simulink model "building_PHPP_v1"  (R2018b)
settings: Solver=ode23s  StartTime=-building.preruntime+8760*3600  StopTime=building.runtime+8760*3600  EnableMultiTasking=on
StartFcn:
  | tic
StopFcn:
  | toc
values from neighbouring files (symbols this model uses):
  A = 7*10*2    (= 140)    [theta_ground_v1.m]    (also in xlswrite1.m = num2cell(data))
  B = A/(0.5 * P)    (= 8.23529411765)    [theta_ground_v1.m]
  building = obj    [BUILDING.m]    (also in create_building_automatic.m = building.save(); ini_building_automatic.m = building.add_variant_hvac(building.variant_hvac, hvac); load_building_automatic.m = building.save())
  C = zeros(1,length(d)+1)    [CONSTRUCTION.m]    (also in DOOR.m = [0 0 0]; WALL.m = [0 0 0]; WINDOW.m = [0 0 0])
  cp = str2num(value)    [CONSTRUCTION.m]
  p = [timevec_weather weather(:,12)]    [BOUNDARY.m]    (also in WEATHER.m = 0; init_carnotUIBK.m = cell2mat(carnotUIBKpaths(i,2)))
  rho = str2num(value)    [CONSTRUCTION.m]    (also in theta_ground_v1.m = 2000)
undefined symbols (not defined in the file or in its folder): Dd, Dreifach, get_building, Qdot_C, Qdot_C_energy, Qdot_H, Qdot_H_energy, Qdot_I_electricity, Qdot_I_electricity_energy, Qdot_I_light, Qdot_I_light_energy, Qdot_I_person, Qdot_I_person_energy, Qdot_S, Qdot_S_energy, Qdot_T_ground, Qdot_T_ground_energy, Qdot_T_neighbour, Qdot_T_neighbour_energy, Qdot_T_opaque, Qdot_T_opaque_energy, Qdot_T_window, Qdot_T_window_energy, Qdot_V_infiltration, Qdot_V_infiltration_energy, Qdot_V_mech, Qdot_V_mech_energy, Qdot_V_window, Qdot_V_window_energy, Tc, Tr, Ts, Wärmeschutzglas, x_CO2, x_H2O, x_VOC
libraries: carnotUIBK x1874, carnot x5, simulink x3
(part 2 of 34)

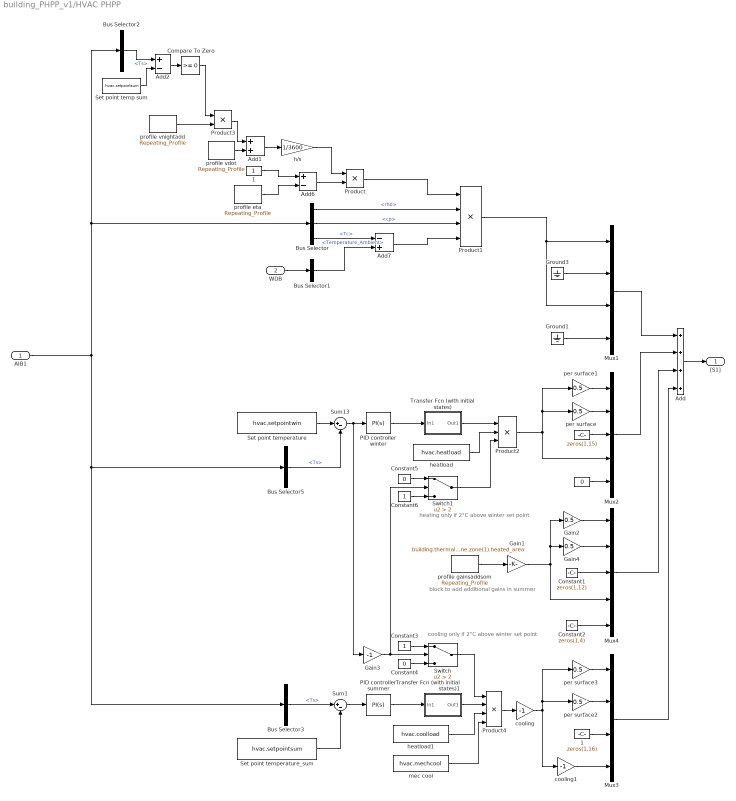
== system building_PHPP_v1/HVAC PHPP ==
  note: cooling only if 2°C above winter set point
  note: block to add additional gains in summer
  note: heating only if 2°C above winter set point
  AIB1 : Inport
  WDB : Inport  Port=2
  " " : Constant  Value=0
  "   " : Constant  Value=zeros(1,15)
  "   1" : Constant  Value=zeros(1,16)
  1 : Constant
  Add : Sum  Inputs=++++
  Add1 : Sum
  Add2 : Sum  Inputs=+-
  Add6 : Sum  Inputs=+-
  Add7 : Sum  Inputs=-+
  Bus Selector : BusSelector  OutputSignals=rho,cp,Tc
  Bus Selector1 : BusSelector  OutputSignals=Temperature_Ambient
  Bus Selector2 : BusSelector  OutputSignals=Ts
  Bus Selector3 : BusSelector  OutputSignals=Ts
  Bus Selector5 : BusSelector  OutputSignals=Ts
  Compare To Zero : simulink/Logic and Bit Operations/Compare To Zero  relop=>=  OutDataTypeStr=boolean
  Constant1 : Constant  Value=zeros(1,12)
  Constant2 : Constant  Value=zeros(1,4)
  Constant3 : Constant
  Constant4 : Constant  Value=0
  Constant5 : Constant  Value=0
  Constant6 : Constant
  Gain1 : Gain  Gain=building.thermalzone.zone(1).heated_area  SaturateOnIntegerOverflow=on  OutDataTypeStr=Inherit: Same as input  ParamDataTypeStr=Inherit: Same as input
  Gain2 : Gain  Gain=0.5  SaturateOnIntegerOverflow=on  OutDataTypeStr=Inherit: Same as input  ParamDataTypeStr=Inherit: Same as input
  Gain3 : Gain  Gain=-1  SaturateOnIntegerOverflow=on  OutDataTypeStr=Inherit: Same as input  ParamDataTypeStr=Inherit: Same as input
  Gain4 : Gain  Gain=0.5  SaturateOnIntegerOverflow=on  OutDataTypeStr=Inherit: Same as input  ParamDataTypeStr=Inherit: Same as input
  Ground1 : Ground
  Ground3 : Ground
  Mux1 : Mux  Inputs=[1 10 1 7]
  Mux2 : Mux  Inputs=[1 1 15 1 1]
  Mux3 : Mux  Inputs=[1 1 16 1]
  Mux4 : Mux  Inputs=[1 1 12 1 4]
  PID controller summer : simulink/Continuous/PID Controller  Controller=PI  Form=Ideal  TimeDomain=Continuous-time  SampleTime=-1  IntegratorMethod=Forward Euler  FilterMethod=Forward Euler  ControllerParametersSource=internal  P=hvac.valves.Kp  I=(1/(hvac.valves.Tn*60))  D=0  UseFilter=on  N=100  TunerSelectOption=Transfer Function Based (PID Tuner App)  InitialConditionSource=internal  InitialConditionForIntegrator=0  InitialConditionForFilter=0  DifferentiatorICPrevScaledInput=0  ExternalReset=none  TrackingMode=off  Kt=1  LimitOutput=on  UpperSaturationLimit=hvac.valves.valve_up  LowerSaturationLimit=hvac.valves.valve_low  LinearizeAsGain=off  AntiWindupMode=clamping  Kb=1  POutMin=[]  POutMax=[]  IOutMin=[]  IOutMax=[]  DOutMin=[]  DOutMax=[]  NOutMin=[]  NOutMax=[]  SumOutMin=[]  SumOutMax=[]  SaturationOutMin=[]  SaturationOutMax=[]  PParamMin=[]  PParamMax=[]  IParamMin=[]  IParamMax=[]  DParamMin=[]  DParamMax=[]  NParamMin=[]  NParamMax=[]  KbParamMin=[]  KbParamMax=[]  KtParamMin=[]  KtParamMax=[]  KbOutMin=[]  KbOutMax=[]  KtOutMin=[]  KtOutMax=[]  IntegratorOutMin=[]  IntegratorOutMax=[]  FilterOutMin=[]  FilterOutMax=[]  SumI1OutMin=[]  SumI1OutMax=[]  SumI2OutMin=[]  SumI2OutMax=[]  SumI3OutMin=[]  SumI3OutMax=[]  SumI4OutMin=[]  SumI4OutMax=[]  SumDOutMin=[]  SumDOutMax=[]  DifferentiatorOutMin=[]  DifferentiatorOutMax=[]  FilterDiffOutCoefMin=[]  FilterDiffOutCoefMax=[]  ReciprocalOutMin=[]  ReciprocalOutMax=[]  SumDenOutMin=[]  SumDenOutMax=[]  SumNumOutMin=[]  SumNumOutMax=[]  DivideOutMin=[]  DivideOutMax=[]  IntegratorContinuousStateAttributes=''  IntegratorStateMustResolveToSignalObject=off  IntegratorRTWStateStorageClass=Auto  FilterContinuousStateAttributes=''  FilterStateMustResolveToSignalObject=off  FilterRTWStateStorageClass=Auto  ParallelPVariant=Passthrough  IdealPVariant=InternalParameters  IVariant=InternalParameters  DVariant=Disabled  IntegratorVariant=Continuous  SatVariant=Enabled  AWVariant=ContClampingIdeal  PCopyVariant=InternalParamsIdeal  TRVariant=Disabled  FdbkBlocksVariant=Forward  IdealPFdbkVariant=Disabled  SatFdbkVariant=Disabled  DerivativeFilterVariant=Disabled  NVariant=Disabled  NCopyVariant=Disabled_SignalSpec  FilterICVariant=Disabled  IntegratorICVariant=InternalICs  ExternalResetVariant=Disabled  TRSumVariant=Passthrough  SumFdbkVariant=Disabled  SumVariant=Sum_PI
  PID controller winter : simulink/Continuous/PID Controller  Controller=PI  Form=Ideal  TimeDomain=Continuous-time  SampleTime=-1  IntegratorMethod=Forward Euler  FilterMethod=Forward Euler  ControllerParametersSource=internal  P=hvac.valves.Kp  I=(1/(hvac.valves.Tn*60))  D=0  UseFilter=on  N=100  TunerSelectOption=Transfer Function Based (PID Tuner App)  InitialConditionSource=internal  InitialConditionForIntegrator=0  InitialConditionForFilter=0  DifferentiatorICPrevScaledInput=0  ExternalReset=none  TrackingMode=off  Kt=1  LimitOutput=on  UpperSaturationLimit=hvac.valves.valve_up  LowerSaturationLimit=hvac.valves.valve_low  LinearizeAsGain=off  AntiWindupMode=clamping  Kb=1  POutMin=[]  POutMax=[]  IOutMin=[]  IOutMax=[]  DOutMin=[]  DOutMax=[]  NOutMin=[]  NOutMax=[]  SumOutMin=[]  SumOutMax=[]  SaturationOutMin=[]  SaturationOutMax=[]  PParamMin=[]  PParamMax=[]  IParamMin=[]  IParamMax=[]  DParamMin=[]  DParamMax=[]  NParamMin=[]  NParamMax=[]  KbParamMin=[]  KbParamMax=[]  KtParamMin=[]  KtParamMax=[]  KbOutMin=[]  KbOutMax=[]  KtOutMin=[]  KtOutMax=[]  IntegratorOutMin=[]  IntegratorOutMax=[]  FilterOutMin=[]  FilterOutMax=[]  SumI1OutMin=[]  SumI1OutMax=[]  SumI2OutMin=[]  SumI2OutMax=[]  SumI3OutMin=[]  SumI3OutMax=[]  SumI4OutMin=[]  SumI4OutMax=[]  SumDOutMin=[]  SumDOutMax=[]  DifferentiatorOutMin=[]  DifferentiatorOutMax=[]  FilterDiffOutCoefMin=[]  FilterDiffOutCoefMax=[]  ReciprocalOutMin=[]  ReciprocalOutMax=[]  SumDenOutMin=[]  SumDenOutMax=[]  SumNumOutMin=[]  SumNumOutMax=[]  DivideOutMin=[]  DivideOutMax=[]  IntegratorContinuousStateAttributes=''  IntegratorStateMustResolveToSignalObject=off  IntegratorRTWStateStorageClass=Auto  FilterContinuousStateAttributes=''  FilterStateMustResolveToSignalObject=off  FilterRTWStateStorageClass=Auto  ParallelPVariant=Passthrough  IdealPVariant=InternalParameters  IVariant=InternalParameters  DVariant=Disabled  IntegratorVariant=Continuous  SatVariant=Enabled  AWVariant=ContClampingIdeal  PCopyVariant=InternalParamsIdeal  TRVariant=Disabled  FdbkBlocksVariant=Forward  IdealPFdbkVariant=Disabled  SatFdbkVariant=Disabled  DerivativeFilterVariant=Disabled  NVariant=Disabled  NCopyVariant=Disabled_SignalSpec  FilterICVariant=Disabled  IntegratorICVariant=InternalICs  ExternalResetVariant=Disabled  TRSumVariant=Passthrough  SumFdbkVariant=Disabled  SumVariant=Sum_PI
  Product : Product
  Product1 : Product  Inputs=4
  Product2 : Product  Inputs=3
  Product3 : Product
  Product4 : Product  Inputs=4
  Set point temp sum : Constant  Value=hvac.setpointsum  VectorParams1D=off
  Set point temperature : Constant  Value=hvac.setpointwin  VectorParams1D=off
  Set point temperature_sum : Constant  Value=hvac.setpointsum  VectorParams1D=off
  Sum1 : Sum  Inputs=|+-
  Sum13 : Sum  Inputs=|+-
  Switch : Switch  Criteria=u2 > Threshold  Threshold=2
  Switch1 : Switch  Criteria=u2 > Threshold  Threshold=2
  Transfer Fcn (with initial states) : Subsystem  mask(Transfer Function with Initial States){N=[1], D=[300  1], X0=0}
      mask prompts: N "Numerator:"; D "Denominator:"; X0 "Initial conditions:"
      mask help: Vector expressions for numerator, and denominator. Coefficients are in descending powers of s.
      mask init:
      | [A,B,C,Dd]=tf2ss(N,D);if (isempty(X0));[m,n]=size(A);X0=zeros(1,m); end;
      mask Help: Specify the initial states for the transfer function.  The state ordering is determined by the m-file tf2ss.  There is no unique mapping of the states in a transfer function to states in a state-space representation.  However, tf2ss will consistently use the same mapping for a given transfer function.
      mask Display: dpoly(N,D,'s')
  Transfer Fcn (with initial states)1 : Subsystem  mask(Transfer Function with Initial States){N=[1], D=[300  1], X0=0}
      mask prompts: N "Numerator:"; D "Denominator:"; X0 "Initial conditions:"
      mask help: Vector expressions for numerator, and denominator. Coefficients are in descending powers of s.
      mask init:
      | [A,B,C,Dd]=tf2ss(N,D);if (isempty(X0));[m,n]=size(A);X0=zeros(1,m); end;
      mask Help: Specify the initial states for the transfer function.  The state ordering is determined by the m-file tf2ss.  There is no unique mapping of the states in a transfer function to states in a state-space representation.  However, tf2ss will consistently use the same mapping for a given transfer function.
      mask Display: dpoly(N,D,'s')
  cooling : Gain  Gain=-1  SaturateOnIntegerOverflow=on  OutDataTypeStr=Inherit: Same as input  ParamDataTypeStr=Inherit: Same as input
  cooling1 : Gain  Gain=-1  SaturateOnIntegerOverflow=on  OutDataTypeStr=Inherit: Same as input  ParamDataTypeStr=Inherit: Same as input
  h/s : Gain  Gain=1/3600
  heatload : Constant  Value=hvac.heatload
  heatload1 : Constant  Value=hvac.coolload
  mec cool : Constant  Value=hvac.mechcool
  per surface{,1..3} (4 alike) : Gain  Gain=0.5  SaturateOnIntegerOverflow=on  OutDataTypeStr=Inherit: Same as input  ParamDataTypeStr=Inherit: Same as input
  profile eta : carnot/Load/General/Repeating_Profile  period=hvac.eta.time(end)  rep_seq_t=hvac.eta.time(1:end-1)  rep_seq_d=hvac.eta.duration  rep_seq_y=hvac.eta.value
  profile gainsaddsom : carnot/Load/General/Repeating_Profile  period=hvac.gainsum.time(end)  rep_seq_t=hvac.gainsum.time(1:end-1)  rep_seq_d=hvac.gainsum.duration  rep_seq_y=hvac.gainsum.value
  profile vdot : carnot/Load/General/Repeating_Profile  period=hvac.vdot_winsom.time(end)  rep_seq_t=hvac.vdot_winsom.time(1:end-1)  rep_seq_d=hvac.vdot_winsom.duration  rep_seq_y=hvac.vdot_winsom.value
  profile vnightadd : carnot/Load/General/Repeating_Profile  period=hvac.night_vent_s.time(end)  rep_seq_t=hvac.night_vent_s.time(1:end-1)  rep_seq_d=hvac.night_vent_s.duration  rep_seq_y=hvac.night_vent_s.value
  "[S1]" : Outport  InitialOutput=0
  wires:
  profile eta/1 -> Add6/2
  profile vdot/1 -> Add1/2
  1/1 -> Add6/1
  Add6/1 -> Product/2
  Product/1 -> Product1/1
  Bus Selector/1 -> Product1/2  "<rho>"
  Bus Selector/2 -> Product1/3  "<cp>"
  Bus Selector/3 -> Add7/1  "<Tc>"
  Product1/1 -> Mux1/3, Mux1/1
  Ground3/1 -> Mux1/2
  WDB/1 -> Bus Selector1/1
  Bus Selector1/1 -> Add7/2  "<Temperature_Ambient>"
  Add7/1 -> Product1/4
  Ground1/1 -> Mux1/4
  h/s/1 -> Product/1
  Add/1 -> "[S1]"/1
  Mux2/1 -> Add/2
  Mux1/1 -> Add/1
  Sum13/1 -> Gain3/1, PID controller winter/1
  Set point temperature/1 -> Sum13/1
  Bus Selector5/1 -> Sum13/2  "<Ts>"
  PID controller winter/1 -> Transfer Fcn (with initial states)/1(In1)
  heatload/1 -> Product2/2
  Product2/1 -> Mux2/4, per surface/1, per surface1/1
  per surface/1 -> Mux2/2
  per surface1/1 -> Mux2/1
  Transfer Fcn (with initial states)/1(Out1) -> Product2/1
  " "/1 -> Mux2/5
  "   "/1 -> Mux2/3
  Add1/1 -> h/s/1
  Product3/1 -> Add1/1
  profile vnightadd/1 -> Product3/2
  Bus Selector2/1 -> Add2/1  "<Ts>"
  Set point temp sum/1 -> Add2/2
  Add2/1 -> Compare To Zero/1
  Compare To Zero/1 -> Product3/1
  Constant2/1 -> Mux4/5
  Constant1/1 -> Mux4/3
  profile gainsaddsom/1 -> Gain1/1
  Gain2/1 -> Mux4/1
  Gain4/1 -> Mux4/2
  Gain1/1 -> Gain2/1, Gain4/1, Mux4/4
  Mux4/1 -> Add/3
  Mux3/1 -> Add/4
  Sum1/1 -> PID controller summer/1
  Set point temperature_sum/1 -> Sum1/2
  Bus Selector3/1 -> Sum1/1  "<Ts>"
  PID controller summer/1 -> Transfer Fcn (with initial states)1/1(In1)
  heatload1/1 -> Product4/3
  Product4/1 -> cooling/1
  per surface2/1 -> Mux3/2
  per surface3/1 -> Mux3/1
  Transfer Fcn (with initial states)1/1(Out1) -> Product4/2
  AIB1/1 -> Bus Selector5/1, Bus Selector3/1, Bus Selector/1, Bus Selector2/1
  "   1"/1 -> Mux3/3
  cooling/1 -> per surface3/1, per surface2/1, cooling1/1
  cooling1/1 -> Mux3/4
  mec cool/1 -> Product4/4
  Constant3/1 -> Switch/1
  Constant4/1 -> Switch/3
  Switch/1 -> Product4/1
  Gain3/1 -> Switch1/2, Switch/2
  Constant5/1 -> Switch1/1
  Constant6/1 -> Switch1/3
  Switch1/1 -> Product2/3

== system building_PHPP_v1/BUILDING/INTERSECTION_1_10 ==
  AIB1 : Inport
  AIB2 : Inport  Port=2
  BDB1 : Inport  Port=3
  BDB2 : Inport  Port=4
  control : Inport  Port=5
  Add : Sum  Inputs=++++++
  Add1 : Sum  Inputs=++++++
  Bus Selector : BusSelector  OutputSignals=Qdot_S
  Bus Selector1 : BusSelector  OutputSignals=Qdot_S
  airexchange_1 : Subsystem  Variant=on  mask{zone=i.matrix_wd, window=1}
      mask prompts: window "wall"
      mask init:
      | if (window <= size(zone,1))
      |     area = zone{window,2};
      |     height = zone{window,14};
      |     inf_C = zone{window,15};
      |     inf_n = zone{window,16};
      |     inf_V = zone{window,17};
      |     control = zone{window,18};
      | else
      |     area = 0;
      |     height = 0;
      |     inf_C = [0 0 0];
      |     inf_n = [0 0 0];
      |     inf_V = [0 0 0];
      |     control = 1;
      | end
      mask Display:
      | fprintf('AIR EXCHANGE\n')
      | %fprintf('\n%s', const.name)
  airexchange_2 : Subsystem  Variant=on  mask{zone=i.matrix_wd, window=2}
      mask prompts: window "wall"
      mask init: same as building_PHPP_v1/BUILDING/INTERSECTION_1_10/airexchange_1
      mask Display:
      | fprintf('AIR EXCHANGE\n')
      | %fprintf('\n%s', const.name)
  airexchange_3 : Subsystem  Variant=on  mask{zone=i.matrix_wd, window=3}
      mask prompts: window "wall"
      mask init: same as building_PHPP_v1/BUILDING/INTERSECTION_1_10/airexchange_1
      mask Display:
      | fprintf('AIR EXCHANGE\n')
      | %fprintf('\n%s', const.name)
  wall_1 : Subsystem  Variant=on  mask{zone=i.matrix_wd, construction=b.construction, wall=1}
      mask init:
      | if (wall <= size(zone,1))
      |     const = construction.get_structure(zone(wall,1))
      |     wallsurface = zone{wall,2};
      |     pos = [zone{wall,4} zone{wall,5} zone{wall,6}];
      |     view_factor = zone{wall,9};
      |     amb_factor = zone{wall,10};
      |     solar_r = zone{wall,11};
      |     solar_ratio1 = solar_r(1);
      |     solar_ratio2 = solar_r(2);
      |     boundary = zone{wall,12};
      |     % still to be implemented with ENABLE, not a VARIANT!
      |     model_ht = zone{wall,8};
      | else
      |     const.name = 'no construction';
      |     wallsurface = 0;
      |     pos = [0 0 0];
      |     view_factor = 0;
      |     amb_factor = 0;
      |     solar_ratio1 = 0;
      |     solar_ratio2 = 0;
      |     boundary = 0;
      |     model_ht = 0;
      | end
      mask Display:
      | fprintf('CONSTRUCTION:\n')
      | fprintf('\n%s', const.name)
  wall_2 : Subsystem  Variant=on  mask{zone=i.matrix_wd, construction=b.construction, wall=2}
      mask init: same as building_PHPP_v1/BUILDING/INTERSECTION_1_10/wall_1
      mask Display:
      | fprintf('CONSTRUCTION:\n')
      | fprintf('\n%s', const.name)
  wall_3 : Subsystem  Variant=on  mask{zone=i.matrix_wd, construction=b.construction, wall=3}
      mask init: same as building_PHPP_v1/BUILDING/INTERSECTION_1_10/wall_1
      mask Display:
      | fprintf('CONSTRUCTION:\n')
      | fprintf('\n%s', const.name)
  S1 : Outport
  S2 : Outport  Port=2
  wires:
  Add/1 -> S1/1
  Add1/1 -> S2/1
  BDB1/1 -> Bus Selector/1
  Bus Selector/1 -> wall_1/3(Qdot_sol1), wall_2/3(Qdot_sol1), wall_3/3(Qdot_sol1)  "<Qdot_S>"
  BDB2/1 -> Bus Selector1/1
  Bus Selector1/1 -> wall_1/4(Qdot_sol2), wall_2/4(Qdot_sol2), wall_3/4(Qdot_sol2)  "<Qdot_S>"
  control/1 -> airexchange_3/3(control), airexchange_2/3(control), airexchange_1/3(control)
  AIB2/1 -> wall_2/2(AIB2), wall_3/2(AIB2), airexchange_3/2(AIB2), airexchange_2/2(AIB2), airexchange_1/2(AIB2), wall_1/2(AIB2)
  AIB1/1 -> wall_2/1(AIB1), wall_3/1(AIB1), airexchange_3/1(AIB1), airexchange_2/1(AIB1), airexchange_1/1(AIB1), wall_1/1(AIB1)
  wall_1/1("[S1]") -> Add/1
  wall_2/1("[S1]") -> Add/2
  wall_3/1("[S1]") -> Add/3
  airexchange_1/1("[S1]") -> Add/4
  airexchange_2/1("[S1]") -> Add/5
  airexchange_3/1("[S1]") -> Add/6
  wall_1/2("[S2]") -> Add1/1
  wall_2/2("[S2]") -> Add1/2
  airexchange_3/2("[S2]") -> Add1/6
  airexchange_2/2("[S2]") -> Add1/5
  airexchange_1/2("[S2]") -> Add1/4
  wall_3/2("[S2]") -> Add1/3

== system building_PHPP_v1/BUILDING/INTERSECTION_1_2 ==
  AIB1 : Inport
  AIB2 : Inport  Port=2
  BDB1 : Inport  Port=3
  BDB2 : Inport  Port=4
  control : Inport  Port=5
  Add : Sum  Inputs=++++++
  Add1 : Sum  Inputs=++++++
  Bus Selector : BusSelector  OutputSignals=Qdot_S
  Bus Selector1 : BusSelector  OutputSignals=Qdot_S
  airexchange_1 : Subsystem  Variant=on  mask{zone=i.matrix_wd, window=1}
      mask prompts: window "wall"
      mask init: same as building_PHPP_v1/BUILDING/INTERSECTION_1_10/airexchange_1
      mask Display:
      | fprintf('AIR EXCHANGE\n')
      | %fprintf('\n%s', const.name)
  airexchange_2 : Subsystem  Variant=on  mask{zone=i.matrix_wd, window=2}
      mask prompts: window "wall"
      mask init: same as building_PHPP_v1/BUILDING/INTERSECTION_1_10/airexchange_1
      mask Display:
      | fprintf('AIR EXCHANGE\n')
      | %fprintf('\n%s', const.name)
  airexchange_3 : Subsystem  Variant=on  mask{zone=i.matrix_wd, window=3}
      mask prompts: window "wall"
      mask init: same as building_PHPP_v1/BUILDING/INTERSECTION_1_10/airexchange_1
      mask Display:
      | fprintf('AIR EXCHANGE\n')
      | %fprintf('\n%s', const.name)
  wall_1 : Subsystem  Variant=on  mask{zone=i.matrix_wd, construction=b.construction, wall=1}
      mask init: same as building_PHPP_v1/BUILDING/INTERSECTION_1_10/wall_1
      mask Display:
      | fprintf('CONSTRUCTION:\n')
      | fprintf('\n%s', const.name)
  wall_2 : Subsystem  Variant=on  mask{zone=i.matrix_wd, construction=b.construction, wall=2}
      mask init: same as building_PHPP_v1/BUILDING/INTERSECTION_1_10/wall_1
      mask Display:
      | fprintf('CONSTRUCTION:\n')
      | fprintf('\n%s', const.name)
  wall_3 : Subsystem  Variant=on  mask{zone=i.matrix_wd, construction=b.construction, wall=3}
      mask init: same as building_PHPP_v1/BUILDING/INTERSECTION_1_10/wall_1
      mask Display:
      | fprintf('CONSTRUCTION:\n')
      | fprintf('\n%s', const.name)
  S1 : Outport
  S2 : Outport  Port=2
  wires:
  Add/1 -> S1/1
  Add1/1 -> S2/1
  BDB1/1 -> Bus Selector/1
  Bus Selector/1 -> wall_1/3(Qdot_sol1), wall_2/3(Qdot_sol1), wall_3/3(Qdot_sol1)  "<Qdot_S>"
  BDB2/1 -> Bus Selector1/1
  Bus Selector1/1 -> wall_1/4(Qdot_sol2), wall_2/4(Qdot_sol2), wall_3/4(Qdot_sol2)  "<Qdot_S>"
  control/1 -> airexchange_3/3(control), airexchange_2/3(control), airexchange_1/3(control)
  AIB2/1 -> wall_2/2(AIB2), wall_3/2(AIB2), airexchange_3/2(AIB2), airexchange_2/2(AIB2), airexchange_1/2(AIB2), wall_1/2(AIB2)
  AIB1/1 -> wall_2/1(AIB1), wall_3/1(AIB1), airexchange_3/1(AIB1), airexchange_2/1(AIB1), airexchange_1/1(AIB1), wall_1/1(AIB1)
  wall_1/1("[S1]") -> Add/1
  wall_2/1("[S1]") -> Add/2
  wall_3/1("[S1]") -> Add/3
  airexchange_1/1("[S1]") -> Add/4
  airexchange_2/1("[S1]") -> Add/5
  airexchange_3/1("[S1]") -> Add/6
  wall_1/2("[S2]") -> Add1/1
  wall_2/2("[S2]") -> Add1/2
  airexchange_3/2("[S2]") -> Add1/6
  airexchange_2/2("[S2]") -> Add1/5
  airexchange_1/2("[S2]") -> Add1/4
  wall_3/2("[S2]") -> Add1/3

== system building_PHPP_v1/BUILDING/INTERSECTION_1_3 ==
  AIB1 : Inport
  AIB2 : Inport  Port=2
  BDB1 : Inport  Port=3
  BDB2 : Inport  Port=4
  control : Inport  Port=5
  Add : Sum  Inputs=++++++
  Add1 : Sum  Inputs=++++++
  Bus Selector : BusSelector  OutputSignals=Qdot_S
  Bus Selector1 : BusSelector  OutputSignals=Qdot_S
  airexchange_1 : Subsystem  Variant=on  mask{zone=i.matrix_wd, window=1}
      mask prompts: window "wall"
      mask init: same as building_PHPP_v1/BUILDING/INTERSECTION_1_10/airexchange_1
      mask Display:
      | fprintf('AIR EXCHANGE\n')
      | %fprintf('\n%s', const.name)
  airexchange_2 : Subsystem  Variant=on  mask{zone=i.matrix_wd, window=2}
      mask prompts: window "wall"
      mask init: same as building_PHPP_v1/BUILDING/INTERSECTION_1_10/airexchange_1
      mask Display:
      | fprintf('AIR EXCHANGE\n')
      | %fprintf('\n%s', const.name)
  airexchange_3 : Subsystem  Variant=on  mask{zone=i.matrix_wd, window=3}
      mask prompts: window "wall"
      mask init: same as building_PHPP_v1/BUILDING/INTERSECTION_1_10/airexchange_1
      mask Display:
      | fprintf('AIR EXCHANGE\n')
      | %fprintf('\n%s', const.name)
  wall_1 : Subsystem  Variant=on  mask{zone=i.matrix_wd, construction=b.construction, wall=1}
      mask init: same as building_PHPP_v1/BUILDING/INTERSECTION_1_10/wall_1
      mask Display:
      | fprintf('CONSTRUCTION:\n')
      | fprintf('\n%s', const.name)
  wall_2 : Subsystem  Variant=on  mask{zone=i.matrix_wd, construction=b.construction, wall=2}
      mask init: same as building_PHPP_v1/BUILDING/INTERSECTION_1_10/wall_1
      mask Display:
      | fprintf('CONSTRUCTION:\n')
      | fprintf('\n%s', const.name)
  wall_3 : Subsystem  Variant=on  mask{zone=i.matrix_wd, construction=b.construction, wall=3}
      mask init: same as building_PHPP_v1/BUILDING/INTERSECTION_1_10/wall_1
      mask Display:
      | fprintf('CONSTRUCTION:\n')
      | fprintf('\n%s', const.name)
  S1 : Outport
  S2 : Outport  Port=2
  wires:
  Add/1 -> S1/1
  Add1/1 -> S2/1
  BDB1/1 -> Bus Selector/1
  Bus Selector/1 -> wall_1/3(Qdot_sol1), wall_2/3(Qdot_sol1), wall_3/3(Qdot_sol1)  "<Qdot_S>"
  BDB2/1 -> Bus Selector1/1
  Bus Selector1/1 -> wall_1/4(Qdot_sol2), wall_2/4(Qdot_sol2), wall_3/4(Qdot_sol2)  "<Qdot_S>"
  control/1 -> airexchange_3/3(control), airexchange_2/3(control), airexchange_1/3(control)
  AIB2/1 -> wall_2/2(AIB2), wall_3/2(AIB2), airexchange_3/2(AIB2), airexchange_2/2(AIB2), airexchange_1/2(AIB2), wall_1/2(AIB2)
  AIB1/1 -> wall_2/1(AIB1), wall_3/1(AIB1), airexchange_3/1(AIB1), airexchange_2/1(AIB1), airexchange_1/1(AIB1), wall_1/1(AIB1)
  wall_1/1("[S1]") -> Add/1
  wall_2/1("[S1]") -> Add/2
  wall_3/1("[S1]") -> Add/3
  airexchange_1/1("[S1]") -> Add/4
  airexchange_2/1("[S1]") -> Add/5
  airexchange_3/1("[S1]") -> Add/6
  wall_1/2("[S2]") -> Add1/1
  wall_2/2("[S2]") -> Add1/2
  airexchange_3/2("[S2]") -> Add1/6
  airexchange_2/2("[S2]") -> Add1/5
  airexchange_1/2("[S2]") -> Add1/4
  wall_3/2("[S2]") -> Add1/3

== system building_PHPP_v1/BUILDING/INTERSECTION_1_4 ==
  AIB1 : Inport
  AIB2 : Inport  Port=2
  BDB1 : Inport  Port=3
  BDB2 : Inport  Port=4
  control : Inport  Port=5
  Add : Sum  Inputs=++++++
  Add1 : Sum  Inputs=++++++
  Bus Selector : BusSelector  OutputSignals=Qdot_S
  Bus Selector1 : BusSelector  OutputSignals=Qdot_S
  airexchange_1 : Subsystem  Variant=on  mask{zone=i.matrix_wd, window=1}
      mask prompts: window "wall"
      mask init: same as building_PHPP_v1/BUILDING/INTERSECTION_1_10/airexchange_1
      mask Display:
      | fprintf('AIR EXCHANGE\n')
      | %fprintf('\n%s', const.name)
  airexchange_2 : Subsystem  Variant=on  mask{zone=i.matrix_wd, window=2}
      mask prompts: window "wall"
      mask init: same as building_PHPP_v1/BUILDING/INTERSECTION_1_10/airexchange_1
      mask Display:
      | fprintf('AIR EXCHANGE\n')
      | %fprintf('\n%s', const.name)
  airexchange_3 : Subsystem  Variant=on  mask{zone=i.matrix_wd, window=3}
      mask prompts: window "wall"
      mask init: same as building_PHPP_v1/BUILDING/INTERSECTION_1_10/airexchange_1
      mask Display:
      | fprintf('AIR EXCHANGE\n')
      | %fprintf('\n%s', const.name)
  wall_1 : Subsystem  Variant=on  mask{zone=i.matrix_wd, construction=b.construction, wall=1}
      mask init: same as building_PHPP_v1/BUILDING/INTERSECTION_1_10/wall_1
      mask Display:
      | fprintf('CONSTRUCTION:\n')
      | fprintf('\n%s', const.name)
  wall_2 : Subsystem  Variant=on  mask{zone=i.matrix_wd, construction=b.construction, wall=2}
      mask init: same as building_PHPP_v1/BUILDING/INTERSECTION_1_10/wall_1
      mask Display:
      | fprintf('CONSTRUCTION:\n')
      | fprintf('\n%s', const.name)
  wall_3 : Subsystem  Variant=on  mask{zone=i.matrix_wd, construction=b.construction, wall=3}
      mask init: same as building_PHPP_v1/BUILDING/INTERSECTION_1_10/wall_1
      mask Display:
      | fprintf('CONSTRUCTION:\n')
      | fprintf('\n%s', const.name)
  S1 : Outport
  S2 : Outport  Port=2
  wires:
  Add/1 -> S1/1
  Add1/1 -> S2/1
  BDB1/1 -> Bus Selector/1
  Bus Selector/1 -> wall_1/3(Qdot_sol1), wall_2/3(Qdot_sol1), wall_3/3(Qdot_sol1)  "<Qdot_S>"
  BDB2/1 -> Bus Selector1/1
  Bus Selector1/1 -> wall_1/4(Qdot_sol2), wall_2/4(Qdot_sol2), wall_3/4(Qdot_sol2)  "<Qdot_S>"
  control/1 -> airexchange_3/3(control), airexchange_2/3(control), airexchange_1/3(control)
  AIB2/1 -> wall_2/2(AIB2), wall_3/2(AIB2), airexchange_3/2(AIB2), airexchange_2/2(AIB2), airexchange_1/2(AIB2), wall_1/2(AIB2)
  AIB1/1 -> wall_2/1(AIB1), wall_3/1(AIB1), airexchange_3/1(AIB1), airexchange_2/1(AIB1), airexchange_1/1(AIB1), wall_1/1(AIB1)
  wall_1/1("[S1]") -> Add/1
  wall_2/1("[S1]") -> Add/2
  wall_3/1("[S1]") -> Add/3
  airexchange_1/1("[S1]") -> Add/4
  airexchange_2/1("[S1]") -> Add/5
  airexchange_3/1("[S1]") -> Add/6
  wall_1/2("[S2]") -> Add1/1
  wall_2/2("[S2]") -> Add1/2
  airexchange_3/2("[S2]") -> Add1/6
  airexchange_2/2("[S2]") -> Add1/5
  airexchange_1/2("[S2]") -> Add1/4
  wall_3/2("[S2]") -> Add1/3

== system building_PHPP_v1/BUILDING/INTERSECTION_1_5 ==
  AIB1 : Inport
  AIB2 : Inport  Port=2
  BDB1 : Inport  Port=3
  BDB2 : Inport  Port=4
  control : Inport  Port=5
  Add : Sum  Inputs=++++++
  Add1 : Sum  Inputs=++++++
  Bus Selector : BusSelector  OutputSignals=Qdot_S
  Bus Selector1 : BusSelector  OutputSignals=Qdot_S
  airexchange_1 : Subsystem  Variant=on  mask{zone=i.matrix_wd, window=1}
      mask prompts: window "wall"
      mask init: same as building_PHPP_v1/BUILDING/INTERSECTION_1_10/airexchange_1
      mask Display:
      | fprintf('AIR EXCHANGE\n')
      | %fprintf('\n%s', const.name)
  airexchange_2 : Subsystem  Variant=on  mask{zone=i.matrix_wd, window=2}
      mask prompts: window "wall"
      mask init: same as building_PHPP_v1/BUILDING/INTERSECTION_1_10/airexchange_1
      mask Display:
      | fprintf('AIR EXCHANGE\n')
      | %fprintf('\n%s', const.name)
  airexchange_3 : Subsystem  Variant=on  mask{zone=i.matrix_wd, window=3}
      mask prompts: window "wall"
      mask init: same as building_PHPP_v1/BUILDING/INTERSECTION_1_10/airexchange_1
      mask Display:
      | fprintf('AIR EXCHANGE\n')
      | %fprintf('\n%s', const.name)
  wall_1 : Subsystem  Variant=on  mask{zone=i.matrix_wd, construction=b.construction, wall=1}
      mask init: same as building_PHPP_v1/BUILDING/INTERSECTION_1_10/wall_1
      mask Display:
      | fprintf('CONSTRUCTION:\n')
      | fprintf('\n%s', const.name)
  wall_2 : Subsystem  Variant=on  mask{zone=i.matrix_wd, construction=b.construction, wall=2}
      mask init: same as building_PHPP_v1/BUILDING/INTERSECTION_1_10/wall_1
      mask Display:
      | fprintf('CONSTRUCTION:\n')
      | fprintf('\n%s', const.name)
  wall_3 : Subsystem  Variant=on  mask{zone=i.matrix_wd, construction=b.construction, wall=3}
      mask init: same as building_PHPP_v1/BUILDING/INTERSECTION_1_10/wall_1
      mask Display:
      | fprintf('CONSTRUCTION:\n')
      | fprintf('\n%s', const.name)
  S1 : Outport
  S2 : Outport  Port=2
  wires:
  Add/1 -> S1/1
  Add1/1 -> S2/1
  BDB1/1 -> Bus Selector/1
  Bus Selector/1 -> wall_1/3(Qdot_sol1), wall_2/3(Qdot_sol1), wall_3/3(Qdot_sol1)  "<Qdot_S>"
  BDB2/1 -> Bus Selector1/1
  Bus Selector1/1 -> wall_1/4(Qdot_sol2), wall_2/4(Qdot_sol2), wall_3/4(Qdot_sol2)  "<Qdot_S>"
  control/1 -> airexchange_3/3(control), airexchange_2/3(control), airexchange_1/3(control)
  AIB2/1 -> wall_2/2(AIB2), wall_3/2(AIB2), airexchange_3/2(AIB2), airexchange_2/2(AIB2), airexchange_1/2(AIB2), wall_1/2(AIB2)
  AIB1/1 -> wall_2/1(AIB1), wall_3/1(AIB1), airexchange_3/1(AIB1), airexchange_2/1(AIB1), airexchange_1/1(AIB1), wall_1/1(AIB1)
  wall_1/1("[S1]") -> Add/1
  wall_2/1("[S1]") -> Add/2
  wall_3/1("[S1]") -> Add/3
  airexchange_1/1("[S1]") -> Add/4
  airexchange_2/1("[S1]") -> Add/5
  airexchange_3/1("[S1]") -> Add/6
  wall_1/2("[S2]") -> Add1/1
  wall_2/2("[S2]") -> Add1/2
  airexchange_3/2("[S2]") -> Add1/6
  airexchange_2/2("[S2]") -> Add1/5
  airexchange_1/2("[S2]") -> Add1/4
  wall_3/2("[S2]") -> Add1/3

== system building_PHPP_v1/BUILDING/INTERSECTION_1_6 ==
  AIB1 : Inport
  AIB2 : Inport  Port=2
  BDB1 : Inport  Port=3
  BDB2 : Inport  Port=4
  control : Inport  Port=5
  Add : Sum  Inputs=++++++
  Add1 : Sum  Inputs=++++++
  Bus Selector : BusSelector  OutputSignals=Qdot_S
  Bus Selector1 : BusSelector  OutputSignals=Qdot_S
  airexchange_1 : Subsystem  Variant=on  mask{zone=i.matrix_wd, window=1}
      mask prompts: window "wall"
      mask init: same as building_PHPP_v1/BUILDING/INTERSECTION_1_10/airexchange_1
      mask Display:
      | fprintf('AIR EXCHANGE\n')
      | %fprintf('\n%s', const.name)
  airexchange_2 : Subsystem  Variant=on  mask{zone=i.matrix_wd, window=2}
      mask prompts: window "wall"
      mask init: same as building_PHPP_v1/BUILDING/INTERSECTION_1_10/airexchange_1
      mask Display:
      | fprintf('AIR EXCHANGE\n')
      | %fprintf('\n%s', const.name)
  airexchange_3 : Subsystem  Variant=on  mask{zone=i.matrix_wd, window=3}
      mask prompts: window "wall"
      mask init: same as building_PHPP_v1/BUILDING/INTERSECTION_1_10/airexchange_1
      mask Display:
      | fprintf('AIR EXCHANGE\n')
      | %fprintf('\n%s', const.name)
  wall_1 : Subsystem  Variant=on  mask{zone=i.matrix_wd, construction=b.construction, wall=1}
      mask init: same as building_PHPP_v1/BUILDING/INTERSECTION_1_10/wall_1
      mask Display:
      | fprintf('CONSTRUCTION:\n')
      | fprintf('\n%s', const.name)
  wall_2 : Subsystem  Variant=on  mask{zone=i.matrix_wd, construction=b.construction, wall=2}
      mask init: same as building_PHPP_v1/BUILDING/INTERSECTION_1_10/wall_1
      mask Display:
      | fprintf('CONSTRUCTION:\n')
      | fprintf('\n%s', const.name)
  wall_3 : Subsystem  Variant=on  mask{zone=i.matrix_wd, construction=b.construction, wall=3}
      mask init: same as building_PHPP_v1/BUILDING/INTERSECTION_1_10/wall_1
      mask Display:
      | fprintf('CONSTRUCTION:\n')
      | fprintf('\n%s', const.name)
  S1 : Outport
  S2 : Outport  Port=2
  wires:
  Add/1 -> S1/1
  Add1/1 -> S2/1
  BDB1/1 -> Bus Selector/1
  Bus Selector/1 -> wall_1/3(Qdot_sol1), wall_2/3(Qdot_sol1), wall_3/3(Qdot_sol1)  "<Qdot_S>"
  BDB2/1 -> Bus Selector1/1
  Bus Selector1/1 -> wall_1/4(Qdot_sol2), wall_2/4(Qdot_sol2), wall_3/4(Qdot_sol2)  "<Qdot_S>"
  control/1 -> airexchange_3/3(control), airexchange_2/3(control), airexchange_1/3(control)
  AIB2/1 -> wall_2/2(AIB2), wall_3/2(AIB2), airexchange_3/2(AIB2), airexchange_2/2(AIB2), airexchange_1/2(AIB2), wall_1/2(AIB2)
  AIB1/1 -> wall_2/1(AIB1), wall_3/1(AIB1), airexchange_3/1(AIB1), airexchange_2/1(AIB1), airexchange_1/1(AIB1), wall_1/1(AIB1)
  wall_1/1("[S1]") -> Add/1
  wall_2/1("[S1]") -> Add/2
  wall_3/1("[S1]") -> Add/3
  airexchange_1/1("[S1]") -> Add/4
  airexchange_2/1("[S1]") -> Add/5
  airexchange_3/1("[S1]") -> Add/6
  wall_1/2("[S2]") -> Add1/1
  wall_2/2("[S2]") -> Add1/2
  airexchange_3/2("[S2]") -> Add1/6
  airexchange_2/2("[S2]") -> Add1/5
  airexchange_1/2("[S2]") -> Add1/4
  wall_3/2("[S2]") -> Add1/3
